simulink model "diagrama_7p21"  (R2021a)
settings: Solver=VariableStepAuto  StartTime=0.0  StopTime=120  RelTol=1e-3
values from neighbouring files (symbols this model uses):
  Af = [0 1 0 0;-n^2 0 0 0;0 0 0 1;0 0 -(2*n)^2 0]    [problema7p21.m]
  Arg = [Arg zeros(6,2) ... (first row only)    [problema7p21.m]
  B2rg = [B2rg;0 0;0 0]    [problema7p21.m]
  Bf = [0;1;0;1]    [problema7p21.m]
  Brg = [Brg;0 0;0 0]    [problema7p21.m]
  K11 = -[K(1,3) K(1,1) K(1,5) K(1,7) K(1,9:12)]    [problema7p21.m]
  K13 = -[K(1,4) K(1,2) K(1,6) K(1,8) K(1,13:16)]    [problema7p21.m]
  K31 = -[K(2,3) K(2,1) K(2,5) K(2,7) K(2,9:12)]    [problema7p21.m]
  K33 = -[K(2,4) K(2,2) K(2,6) K(2,8) K(2,13:16)]    [problema7p21.m]
  phi0 = 1*pi/180    (= 0.0174532925199)    [problema7p21.m]
  psi0 = 1*pi/180    (= 0.0174532925199)    [problema7p21.m]
  wx0 = 0.001*pi/180    (= 1.74532925199e-05)    [problema7p21.m]
  wz0 = 0.001*pi/180    (= 1.74532925199e-05)    [problema7p21.m]
settings Model: Creator=willi  LastModifiedBy=willi

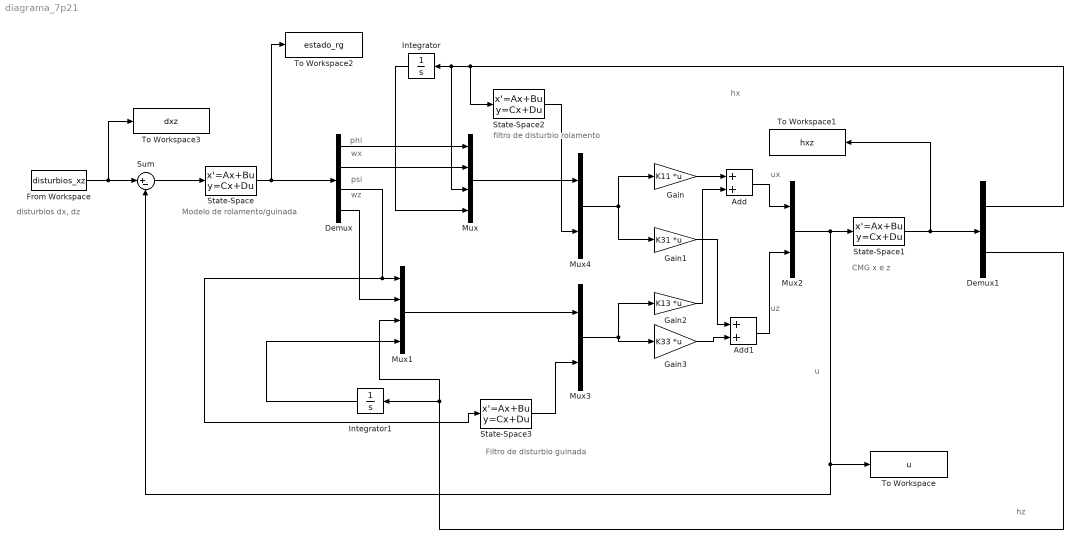
== system diagrama_7p21 ==
  note: Filtro de
      | disturbio
      | guinada
  note: filtro de
      | disturbio
      | rolamento
  note: disturbios dx, dz
  note: phi
  note: CMG x e z
  note: psi
  note: u
  note: ux
  note: wx
  note: wz
  note: Modelo de
      | rolamento/guinada
  note: hx
  note: hz
  note: uz
  Add : Sum
  Add1 : Sum
  Demux : Demux
  Demux1 : Demux  Outputs=2
  From Workspace : FromWorkspace  VariableName=disturbios_xz
  Gain : Gain  Gain=K11  Multiplication=Matrix(K*u)
  Gain1 : Gain  Gain=K31  Multiplication=Matrix(K*u)
  Gain2 : Gain  Gain=K13  Multiplication=Matrix(K*u)
  Gain3 : Gain  Gain=K33  Multiplication=Matrix(K*u)
  Integrator : Integrator
  Integrator1 : Integrator
  Mux : Mux
  Mux1 : Mux
  Mux2 : Mux  Inputs=2
  Mux3 : Mux  Inputs=2
  Mux4 : Mux  Inputs=2
  State-Space : StateSpace  A=Arg(1:4,1:4)  B=B2rg(1:4,:)  C=[0 0 1 0;1 0 0 0;0 0 0 1;0 1 0 0]  D=zeros(4,2)  InitialCondition=[wx0;wz0;phi0;psi0]
  State-Space1 : StateSpace  A=Arg(5:6,5:6)  B=Brg(5:6,:)  C=eye(2,2)  D=zeros(2,2)  InitialCondition=[0;0]
  State-Space2 : StateSpace  A=Af  B=Bf  C=[1 0 0 0;0 1 0 0;0 0 1 0;0 0 0 1]  D=[0;0;0;0]  InitialCondition=-1
  State-Space3 : StateSpace  A=Af  B=Bf  C=[1 0 0 0;0 1 0 0;0 0 1 0;0 0 0 1]  D=[0;0;0;0]  InitialCondition=-1
  Sum : Sum  Inputs=|+-
  To Workspace : ToWorkspace  VariableName=u  SaveFormat=Structure With Time  SampleTime=-1
  To Workspace1 : ToWorkspace  VariableName=hxz  SaveFormat=Structure With Time  SampleTime=-1
  To Workspace2 : ToWorkspace  VariableName=estado_rg  SaveFormat=Structure With Time  SampleTime=-1
  To Workspace3 : ToWorkspace  VariableName=dxz  SaveFormat=Structure With Time  SampleTime=-1
  wires:
  Add/1 -> Mux2/1
  Gain/1 -> Add/1
  Gain3/1 -> Add1/2
  Gain1/1 -> Add1/1
  Add1/1 -> Mux2/2
  Demux/1 -> Mux/1
  Integrator/1 -> Mux/4
  Gain2/1 -> Add/2
  Demux/2 -> Mux/2
  Demux/3 -> State-Space3/1, Mux1/1
  State-Space/1 -> To Workspace2/1, Demux/1
  Integrator1/1 -> Mux1/4
  Sum/1 -> State-Space/1
  From Workspace/1 -> To Workspace3/1, Sum/1
  Demux1/2 -> Mux1/3, Integrator1/1
  Mux2/1 -> State-Space1/1, Sum/2, To Workspace/1
  State-Space1/1 -> Demux1/1, To Workspace1/1
  Demux1/1 -> State-Space2/1, Mux/3, Integrator/1
  Demux/4 -> Mux1/2
  Mux1/1 -> Mux3/1
  Mux/1 -> Mux4/1
  State-Space2/1 -> Mux4/2
  Mux4/1 -> Gain1/1, Gain/1
  Mux3/1 -> Gain2/1, Gain3/1
  State-Space3/1 -> Mux3/2
